simulink model "slcp1"  (Simulink 4.00)
settings: Solver=ode45  SolverMode=SingleTasking  StartTime=0.0  StopTime=1000  MaxStep=0.1  RelTol=1e-3  AbsTol=1e-6
PreLoadFcn:
  | initcp1
libraries: fuzblock x1
CloseFcn:
  | AnimFigTitle = [winName, ': Cart & Pole Animation']; AnimFigH = findobj(0,'Name',AnimFigTitle); close(AnimFigH)
settings Model: CovMetricSettings=d  Creator=pascal  LastModifiedBy=nhickey  SaveTime=off  SaveOutput=off  LimitDataPoints=off  RTWTemplateMakefile=grt_unix.tmf  TryForceingSFcnDF=off  ExtModeTrigMode=oneshot  BlockReductionOpt=off

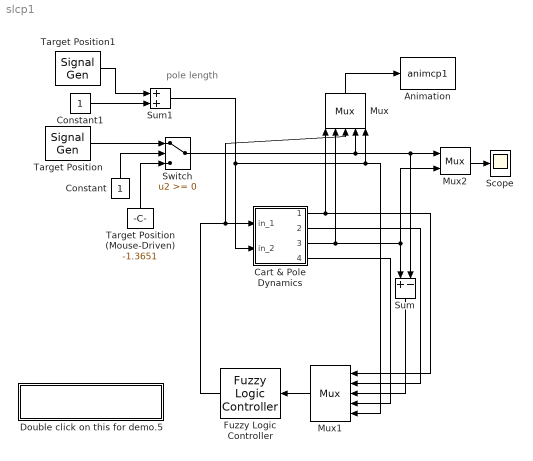
== system slcp1 ==
  note: pole
      | length
  Animation : S-Function  FunctionName=animcp1  PortCounts=[]  SFunctionModules=''
  Cart & Pole Dynamics : Subsystem  mask(Cart & Pole){@1=[0, 0, 0, 0], @2=[1.0, 9.8]}
      mask prompts: @1 "Initial Conditions (angle, angular velocity, cart position and cart velocity):"; @2 "Physical Specifications (cart mass and g):"
      mask help: Inverted Pendulum (cart & pole)
      mask init:
      | init_cond = @1; spec = @2;mc=spec(1);g=spec(2);
      settings: RTWFcnNameOpts=Auto  RTWFileNameOpts=Auto
      mask Help: Inverted Pendulum
      mask Display: plot(-4,-1,4,6,[0 3 2.8 -0.2 0],[1 5 5.15 1.15 1],[-1 -1 1 1 -1],[1 0 0 1 1],[-3.5 3.5],[0 0])
  Constant : Constant  Orientation=up  Value=1
  Constant1 : Constant  Value=1
  Double click on this for demo.5 : Subsystem
      settings: OpenFcn=initcp  RTWFcnNameOpts=Auto  RTWFileNameOpts=Auto
      mask Display: disp('Variable Initialization')
  Fuzzy Logic Controller : fuzblock/Fuzzy Logic  Controller  Orientation=left  fis=fismat
  Mux : Mux  Orientation=up  Inputs=5  BusCreatorMode=off
      settings: DisplayOption=none
  Mux1 : Mux  Orientation=left  Inputs=5  BusCreatorMode=off
      settings: DisplayOption=none
  Mux2 : Mux  Inputs=2  BusCreatorMode=off
      settings: DisplayOption=none
  Scope : Scope
      settings: TickLabels=on  TimeRange=10.000000  YMin=-2.000000  YMax=2.000000  SaveToWorkspace=off  SaveName=ScopeData  DataFormat=Array  LimitDataPoints=on  MaxDataPoints=5000
  Sum : Sum  Orientation=down  Inputs=+-  SaturateOnIntegerOverflow=on
  Sum1 : Sum  Inputs=++  SaturateOnIntegerOverflow=on
  Switch : Switch  Threshold=0
  Target Position : SignalGenerator  WaveForm=sawtooth  Amplitude=1.500000  Frequency=0.628320  Units=rad/sec
  Target Position (Mouse-Driven) : Constant  Orientation=up  Value=-1.3651
  Target Position1 : SignalGenerator  WaveForm=sine  Amplitude=0.500000  Frequency=6.000000  Units=rad/sec
  wires:
  Mux1/1 -> Fuzzy Logic Controller/1
  Sum/1 -> Mux1/3
  Cart & Pole Dynamics/2(out_2) -> Mux1/2
  Cart & Pole Dynamics/1(out_1) -> Mux1/1, Mux/1
  Cart & Pole Dynamics/3(out_3) -> Mux/2, Sum/1, Mux2/2
  Fuzzy Logic Controller/1 -> Cart & Pole Dynamics/1(in_1), Mux/3
  Switch/1 -> Mux/4, Sum/2, Mux2/1
  Cart & Pole Dynamics/4(out_4) -> Mux1/4
  Mux/1 -> Animation/1
  Mux2/1 -> Scope/1
  Target Position (Mouse-Driven)/1 -> Switch/3
  Constant/1 -> Switch/2
  Target Position/1 -> Switch/1
  Sum1/1 -> Cart & Pole Dynamics/2(in_2), Mux/5, Mux1/5
  Target Position1/1 -> Sum1/1
  Constant1/1 -> Sum1/2

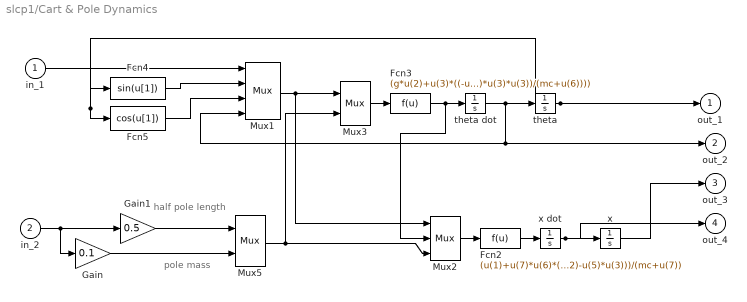
== system slcp1/Cart & Pole Dynamics ==
  note: half pole length
  note: pole mass
  in_1 : Inport  Port=1
  in_2 : Inport  Port=2
  Fcn2 : Fcn  Expr=(u(1)+u(7)*u(6)*(u(4)*u(4)*u(2)-u(5)*u(3)))/(mc+u(7))
  Fcn3 : Fcn  Expr=(g*u(2)+u(3)*((-u(1)-u(6)*u(5)*u(4)*u(4)*u(2))/(mc+u(6))))/(u(5)*(4/3-(u(6)*u(3)*u(3))/(mc+u(6))))
  Fcn4 : Fcn  Expr=sin(u[1])
  Fcn5 : Fcn  Expr=cos(u[1])
  Gain : Gain  Gain=0.1  Multiplication=Element-wise(K.*u)  SaturateOnIntegerOverflow=on
  Gain1 : Gain  Gain=0.5  Multiplication=Element-wise(K.*u)  SaturateOnIntegerOverflow=on
  Mux1 : Mux  Inputs=4  BusCreatorMode=off
      settings: DisplayOption=none
  Mux2 : Mux  Inputs=[4,1,2]  BusCreatorMode=off
      settings: DisplayOption=none
  Mux3 : Mux  Inputs=[4,2]  BusCreatorMode=off
      settings: DisplayOption=none
  Mux5 : Mux  Inputs=2  BusCreatorMode=off
      settings: DisplayOption=none
  theta : Integrator  ExternalReset=none  InitialConditionSource=internal  InitialCondition=init_cond(1)  LimitOutput=off  UpperSaturationLimit=inf  LowerSaturationLimit=-inf  ShowSaturationPort=off  ShowStatePort=off  AbsoluteTolerance=auto
  theta dot : Integrator  ExternalReset=none  InitialConditionSource=internal  InitialCondition=init_cond(2)  LimitOutput=off  UpperSaturationLimit=inf  LowerSaturationLimit=-inf  ShowSaturationPort=off  ShowStatePort=off  AbsoluteTolerance=auto
  x : Integrator  ExternalReset=none  InitialConditionSource=internal  InitialCondition=init_cond(3)  LimitOutput=off  UpperSaturationLimit=inf  LowerSaturationLimit=-inf  ShowSaturationPort=off  ShowStatePort=off  AbsoluteTolerance=auto
  x dot : Integrator  ExternalReset=none  InitialConditionSource=internal  InitialCondition=init_cond(4)  LimitOutput=off  UpperSaturationLimit=inf  LowerSaturationLimit=-inf  ShowSaturationPort=off  ShowStatePort=off  AbsoluteTolerance=auto
  out_1 : Outport  Port=1  InitialOutput=0
  out_2 : Outport  Port=2  InitialOutput=0
  out_3 : Outport  Port=3  InitialOutput=0
  out_4 : Outport  Port=4  InitialOutput=0
  wires:
  theta/1 -> out_1/1, Fcn5/1, Fcn4/1
  Fcn5/1 -> Mux1/3
  Fcn4/1 -> Mux1/2
  theta dot/1 -> theta/1, out_2/1, Mux1/4
  Fcn3/1 -> theta dot/1, Mux2/2
  Fcn2/1 -> x dot/1
  Mux2/1 -> Fcn2/1
  x dot/1 -> x/1, out_4/1
  x/1 -> out_3/1
  in_1/1 -> Mux1/1
  Mux3/1 -> Fcn3/1
  Mux1/1 -> Mux2/1, Mux3/1
  Gain/1 -> Mux5/2
  Mux5/1 -> Mux3/2, Mux2/3
  in_2/1 -> Gain/1, Gain1/1
  Gain1/1 -> Mux5/1

== system slcp1/Double click on this for demo.5 ==
